simulink model "cps_medium_network_v2"  (R2012b)
settings: Solver=FixedStepDiscrete  StartTime=0.0  StopTime=8.5  RelTol=20e-5
model workspace (MAT data in the model file):
  ini_block_hpos = -0.4
  ini_block_vpos = 0.11
  ini_nozzle_vpos = 0.3
settings Model: Creator=pmosterm  LastModifiedBy=pmosterm
settings SolverCC: ZcThreshold=2e-5  MaxConsecutiveZCs=20  EnableConcurrentExecution=on  ConcurrentTasks=on  ZeroCrossAlgorithm=Adaptive  SolverResetMethod=Robust
settings DataIOCC: SignalLoggingSaveFormat=ModelDataLogs
settings OptimizationCC: InlineParams=on
settings DebuggingCC: ReadBeforeWriteMsg=DisableAll  WriteAfterWriteMsg=DisableAll  WriteAfterReadMsg=DisableAll  AlgebraicLoopMsg=error  UnderspecifiedInitializationDetection=Simplified  FcnCallInpInsideContextMsg=EnableAllAsWarning  ModelReferenceExtraNoncontSigs=warning
settings ModelReferenceCC: ModelReferenceNumInstancesAllowed=Single
settings GRTTargetCC: CombineOutputUpdateFcns=off  GRTInterface=on
settings ConfigurationSet: Description=SimMechanics 2G

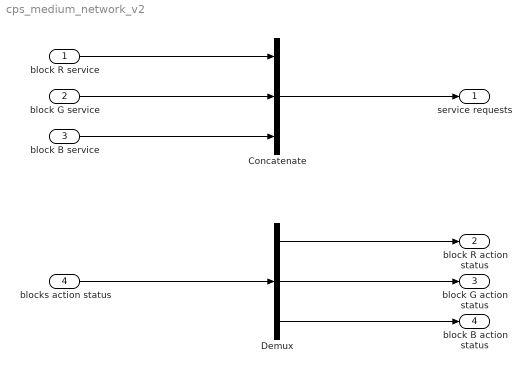
== system cps_medium_network_v2 ==
  block R service : Inport  OutDataTypeStr=Bus: slBusBlockOps  BusOutputAsStruct=on
  block G service : Inport  Port=2  OutDataTypeStr=Bus: slBusBlockOps  BusOutputAsStruct=on
  block B service : Inport  Port=3  OutDataTypeStr=Bus: slBusBlockOps  BusOutputAsStruct=on
  blocks action status : Inport  Port=4
  Concatenate : Concatenate  NumInputs=3
  Demux : Demux  Outputs=3
  service requests : Outport  OutDataTypeStr=Bus: slBusBlockOps  PortDimensions=3  BusOutputAsStruct=on
  block R action status : Outport  Port=2
  block G action status : Outport  Port=3
  block B action status : Outport  Port=4
  wires:
  Demux/1 -> block R action status/1
  Concatenate/1 -> service requests/1
  block G service/1 -> Concatenate/2
  blocks action status/1 -> Demux/1
  Demux/2 -> block G action status/1
  block R service/1 -> Concatenate/1
  block B service/1 -> Concatenate/3
  Demux/3 -> block B action status/1
